simulink model "Ident_Validacao"  (R2015a)
settings: Solver=ode45  StartTime=0.0  StopTime=t(end)  RelTol=1e-3
values from neighbouring files (symbols this model uses):
  T = 0.04    [Ident_RLtool.m]
  Y1 = tf( [-0.0001849 0.601 4.177], [1 -0.5356 0.1912 -0.06649], T )    [Ident_RLtool.m]
  Y2 = tf( [0.0003743 1.097 6.9], [1 -0.4647 0.1618 -0.04697], T )    [Ident_RLtool.m]
  Y3 = tf( [0.001112 0.9936 5.355], [1 -0.469 0.182 -0.05863], T )    [Ident_RLtool.m]
settings Model: Creator=Lucas  LastModifiedBy=Lucas

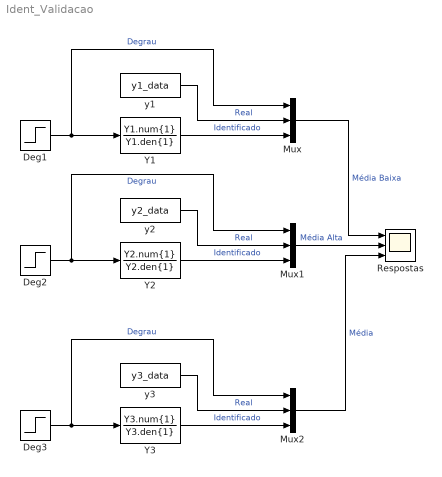
== system Ident_Validacao ==
  Deg1 : Step  Time=6*T  After=10  SampleTime=T
  Deg2 : Step  Time=6*T  After=10  SampleTime=T
  Deg3 : Step  Time=6*T  After=10  SampleTime=T
  Mux : Mux  Inputs=3
  Mux1 : Mux  Inputs=3
  Mux2 : Mux  Inputs=3
  Respostas : Scope  NumInputPorts=3
      settings: ShowLegends=on  YMin=-5~-5~-5  YMax=5~5~5
  Y1 : DiscreteTransferFcn  Numerator=Y1.num{1}  Denominator=Y1.den{1}  SampleTime=T
  Y2 : DiscreteTransferFcn  Numerator=Y2.num{1}  Denominator=Y2.den{1}  SampleTime=T
  Y3 : DiscreteTransferFcn  Numerator=Y3.num{1}  Denominator=Y3.den{1}  SampleTime=T
  y1 : FromWorkspace  VariableName=y1_data  SampleTime=T
  y2 : FromWorkspace  VariableName=y2_data  SampleTime=T
  y3 : FromWorkspace  VariableName=y3_data  SampleTime=T
  wires:
  Mux/1 -> Respostas/1  "Média Baixa"
  Y1/1 -> Mux/3  "Identificado"
  Deg1/1 -> Mux/1, Y1/1  "Degrau"
  y1/1 -> Mux/2  "Real"
  Y2/1 -> Mux1/3  "Identificado"
  Deg2/1 -> Y2/1, Mux1/1  "Degrau"
  y2/1 -> Mux1/2  "Real"
  Y3/1 -> Mux2/3  "Identificado"
  Deg3/1 -> Mux2/1, Y3/1  "Degrau"
  y3/1 -> Mux2/2  "Real"
  Mux2/1 -> Respostas/3  "Média"
  Mux1/1 -> Respostas/2  "Média Alta"
